simulink model "old_FMS"  (R2018b)
settings: configuration reference "FMS_config" (kept outside this file)
undefined symbols (not defined in the file): actuator_cmd, DiscIntNeverNeededParam, FMS_EXPORT, FMS_PARAM, mode, p_cmd, phi_cmd, psi_rate_cmd, q_cmd, r_cmd, reset, state, theta_cmd, throttle_cmd, timestamp, u_cmd, v_cmd, w_cmd
libraries: simulink x39, Rotation x2, Filter x1
(part 1 of 2)
settings Model: Creator=zouji  LastModifiedBy=zouji
settings ConfigSetRef: SourceLocation=Base Workspace

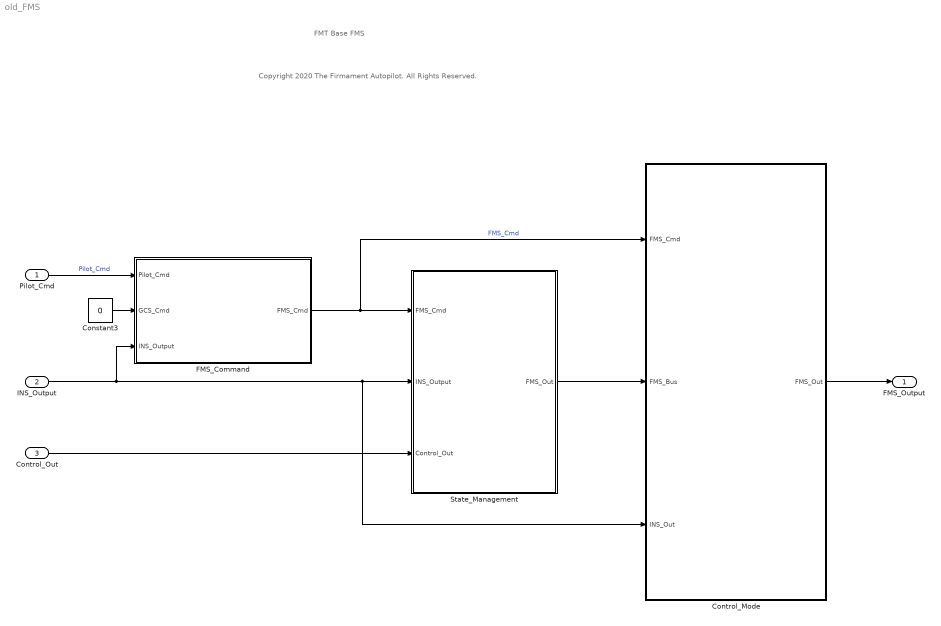
== system old_FMS ==
  note: FMT Base FMS
  note: Copyright 2020 The Firmament Autopilot. All Rights Reserved.
  Pilot_Cmd : Inport  OutDataTypeStr=Bus: Pilot_Cmd_Bus
  INS_Output : Inport  Port=2  OutDataTypeStr=Bus: INS_Out_Bus
  Control_Out : Inport  Port=3  OutDataTypeStr=Bus: Control_Out_Bus
  Constant3 : Constant  Value=0
  Control_Mode : Subsystem
  FMS_Command : Subsystem
  State_Management : Subsystem
  FMS_Output : Outport  OutDataTypeStr=Bus: FMS_Out_Bus
  wires:
  Control_Mode/1(FMS_Out) -> FMS_Output/1
  INS_Output/1 -> FMS_Command/3(INS_Output), Control_Mode/3(INS_Out), State_Management/2(INS_Output)
  Pilot_Cmd/1 -> FMS_Command/1(Pilot_Cmd)  "Pilot_Cmd"
  Constant3/1 -> FMS_Command/2(GCS_Cmd)
  FMS_Command/1(FMS_Cmd) -> Control_Mode/1(FMS_Cmd), State_Management/1(FMS_Cmd)  "FMS_Cmd"
  State_Management/1(FMS_Out) -> Control_Mode/2(FMS_Bus)
  Control_Out/1 -> State_Management/3(Control_Out)

== system old_FMS/Control_Mode ==
  FMS_Cmd : Inport
  FMS_Bus : Inport  Port=2
  INS_Out : Inport  Port=3
  Acro_Mode : Subsystem  TreatAsAtomicUnit=on
  Altitude_Hold_Mode : Subsystem  TreatAsAtomicUnit=on
  Bus Selector : BusSelector  OutputSignals=flag
  Bus Selector1 : BusSelector  OutputSignals=mode
  Manual_Mode : Subsystem  TreatAsAtomicUnit=on
  Merge : Merge  Inputs=5
  Mode_Logic : Stateflow chart  TreatAsAtomicUnit=on
  Position_Mode : Subsystem  TreatAsAtomicUnit=on
  Switch Case : SwitchCase  CaseConditions={2,3,4,5}
  Unknown_Mode : Subsystem  TreatAsAtomicUnit=on
  FMS_Out : Outport
  wires:
  INS_Out/1 -> Manual_Mode/2(INS_Out), Altitude_Hold_Mode/2(INS_Out), Position_Mode/2(INS_Out), Bus Selector/1
  FMS_Cmd/1 -> Bus Selector1/1, Manual_Mode/1(FMS_Cmd), Acro_Mode/2(FMS_Cmd), Altitude_Hold_Mode/1(FMS_Cmd), Position_Mode/1(FMS_Cmd)
  Switch Case/1 -> Position_Mode/Action
  Position_Mode/1(FMS_Out) -> Merge/1
  Switch Case/5 -> Unknown_Mode/Action
  Bus Selector/1 -> Mode_Logic/2(flag)  "<flag>"
  Merge/1 -> FMS_Out/1
  Unknown_Mode/1(FMS_Out) -> Merge/5
  FMS_Bus/1 -> Unknown_Mode/1(FMS_Bus), Acro_Mode/1(FMS_Bus), Manual_Mode/3(FMS_Bus), Altitude_Hold_Mode/3(FMS_Bus), Position_Mode/3(FMS_Bus)
  Bus Selector1/1 -> Mode_Logic/1(mode)  "<mode>"
  Mode_Logic/1(control_mode) -> Switch Case/1  "control_mode"
  Switch Case/2 -> Altitude_Hold_Mode/Action
  Altitude_Hold_Mode/1(FMS_Out) -> Merge/2
  Switch Case/3 -> Manual_Mode/Action
  Manual_Mode/1(FMS_Out) -> Merge/3
  Acro_Mode/1(FMS_Out) -> Merge/4
  Switch Case/4 -> Acro_Mode/Action

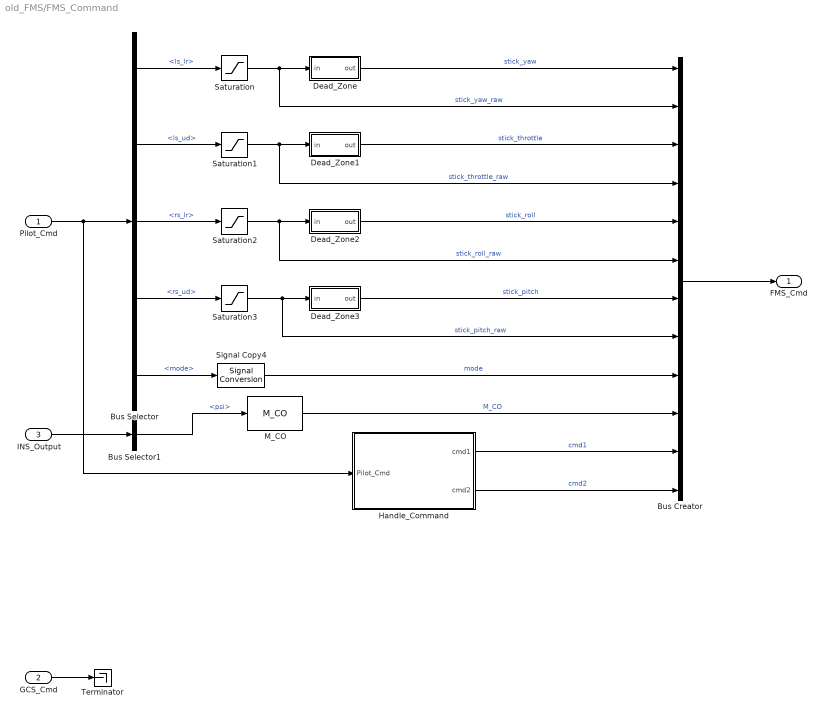
== system old_FMS/FMS_Command ==
  Pilot_Cmd : Inport
  GCS_Cmd : Inport  Port=2
  INS_Output : Inport  Port=3
  Bus Creator : BusCreator  Inputs=12
  Bus Selector : BusSelector  OutputSignals=ls_lr,ls_ud,rs_lr,rs_ud,mode
  Bus Selector1 : BusSelector  OutputSignals=psi
  Dead_Zone : Subsystem  mask{len=FMS_PARAM.StickDeadZone}
      mask prompts: len "Zone Half Length"
  Dead_Zone1 : Subsystem  mask{len=FMS_PARAM.StickDeadZone}
      mask prompts: len "Zone Half Length"
  Dead_Zone2 : Subsystem  mask{len=FMS_PARAM.StickDeadZone}
      mask prompts: len "Zone Half Length"
  Dead_Zone3 : Subsystem  mask{len=FMS_PARAM.StickDeadZone}
      mask prompts: len "Zone Half Length"
  Handle_Command : Subsystem
  M_CO : Rotation/M_CO  SystemSampleTime=-1
  Saturation{,1..3} (4 alike) : Saturate  UpperLimit=1  LowerLimit=-1
  Signal Copy4 : SignalConversion  OverrideOpt=off
  Terminator : Terminator
  FMS_Cmd : Outport
  wires:
  GCS_Cmd/1 -> Terminator/1
  Pilot_Cmd/1 -> Handle_Command/1(Pilot_Cmd), Bus Selector/1
  Bus Selector/1 -> Saturation/1  "<ls_lr>"
  Bus Selector/2 -> Saturation1/1  "<ls_ud>"
  Bus Selector/3 -> Saturation2/1  "<rs_lr>"
  Bus Selector/4 -> Saturation3/1  "<rs_ud>"
  Bus Selector/5 -> Signal Copy4/1  "<mode>"
  Saturation/1 -> Bus Creator/2, Dead_Zone/1(in)  "stick_yaw_raw"
  Saturation1/1 -> Bus Creator/4, Dead_Zone1/1(in)  "stick_throttle_raw"
  Saturation2/1 -> Bus Creator/6, Dead_Zone2/1(in)  "stick_roll_raw"
  Saturation3/1 -> Bus Creator/8, Dead_Zone3/1(in)  "stick_pitch_raw"
  Signal Copy4/1 -> Bus Creator/9  "mode"
  Bus Creator/1 -> FMS_Cmd/1
  Dead_Zone/1(out) -> Bus Creator/1  "stick_yaw"
  Dead_Zone1/1(out) -> Bus Creator/3  "stick_throttle"
  Dead_Zone2/1(out) -> Bus Creator/5  "stick_roll"
  Dead_Zone3/1(out) -> Bus Creator/7  "stick_pitch"
  INS_Output/1 -> Bus Selector1/1
  Bus Selector1/1 -> M_CO/1  "<psi>"
  M_CO/1 -> Bus Creator/10  "M_CO"
  Handle_Command/1(cmd1) -> Bus Creator/11  "cmd1"
  Handle_Command/2(cmd2) -> Bus Creator/12  "cmd2"

== system old_FMS/State_Management ==
  FMS_Cmd : Inport
  INS_Output : Inport  Port=2
  Control_Out : Inport  Port=3
  Arm_Event : Subsystem
  "Arm_Prerequisite " : Subsystem
      settings: MinAlgLoopOccurrences=on
  Bus Assignment : BusAssignment  AssignedSignals=actuator_cmd,state,reset,timestamp
  Bus Selector : BusSelector  OutputSignals=cmd1.cmd1_force_disarm,cmd2.cmd2_test_motor
  Compare To Constant : simulink/Logic and Bit Operations/Compare To Constant  relop=<  const=2  OutDataTypeStr=uint8
  Constant : Constant  Value=0  OutDataTypeStr=Bus: FMS_Out_Bus
  Delay : Delay  DelayLength=1
  State_Logic : Stateflow chart  TreatAsAtomicUnit=on
  Subsystem : Subsystem
  timestamp : Subsystem  mask{sample_time=FMS_EXPORT.period}
      mask prompts: sample_time "sample time (ms)"
  FMS_Out : Outport
  wires:
  Constant/1 -> Bus Assignment/1
  Bus Assignment/1 -> FMS_Out/1
  Arm_Event/2(disarm_event) -> State_Logic/4(Disarm_Event)
  Arm_Event/1(arm_event) -> State_Logic/3(Arm_Event)
  FMS_Cmd/1 -> Bus Selector/1, Arm_Event/2(FMS_Cmd)
  "Arm_Prerequisite "/2(Disarm_Allowed) -> State_Logic/2(Disarm_Allowed)
  "Arm_Prerequisite "/1(Arm_Allowed) -> State_Logic/1(Arm_Allowed)
  INS_Output/1 -> Arm_Event/1(INS_Output), "Arm_Prerequisite "/1(INS_Output)
  State_Logic/1(PWM_Cmd) -> Subsystem/1(pwm_in)
  Subsystem/1(pwm_out) -> Bus Assignment/2
  State_Logic/2(State) -> Delay/1, Compare To Constant/1, Bus Assignment/3
  Compare To Constant/1 -> Bus Assignment/4
  Arm_Event/3(Stick_Throttle) -> State_Logic/5(Stick_Throttle)
  timestamp/1(timestamp_ms) -> Bus Assignment/5
  Control_Out/1 -> Arm_Event/3(Control_Out)
  Delay/1 -> Arm_Event/4(State)
  Bus Selector/1 -> State_Logic/6(Force_Disarm)  "<cmd1_force_disarm>"
  Bus Selector/2 -> State_Logic/7(Test_Motor)  "<cmd2_test_motor>"

== system old_FMS/Control_Mode/Acro_Mode ==
  FMS_Bus : Inport
  FMS_Cmd : Inport  Port=2
  Action Port : ActionPort  InitializeStates=reset  ActionType=case
  Bus Assignment : BusAssignment  AssignedSignals=mode,throttle_cmd,p_cmd,q_cmd,r_cmd
  Command_Generator : Subsystem
  Constant : Constant  Value=5  OutDataTypeStr=Inherit: Inherit via back propagation
  FMS_Out : Outport
  wires:
  Bus Assignment/1 -> FMS_Out/1
  Constant/1 -> Bus Assignment/2
  FMS_Bus/1 -> Bus Assignment/1
  Command_Generator/1(throttle_cmd) -> Bus Assignment/3
  Command_Generator/2(p_cmd_radPs) -> Bus Assignment/4
  Command_Generator/3(q_cmd_radPs) -> Bus Assignment/5
  Command_Generator/4(r_cmd_radPs) -> Bus Assignment/6
  FMS_Cmd/1 -> Command_Generator/1(FMS_Cmd)

== system old_FMS/Control_Mode/Altitude_Hold_Mode ==
  FMS_Cmd : Inport
  INS_Out : Inport  Port=2
  FMS_Bus : Inport  Port=3
  Action Port : ActionPort  InitializeStates=reset  ActionType=case
  Bus Assignment : BusAssignment  AssignedSignals=mode,phi_cmd,theta_cmd,w_cmd,psi_rate_cmd
  Command_Generator : Subsystem
  Constant : Constant  Value=3  OutDataTypeStr=Inherit: Inherit via back propagation
  FMS_Out : Outport
  wires:
  FMS_Cmd/1 -> Command_Generator/3(FMS_Cmd)
  FMS_Bus/1 -> Command_Generator/1(FMS_Out), Bus Assignment/1
  Constant/1 -> Bus Assignment/2
  INS_Out/1 -> Command_Generator/2(INS_Out)
  Bus Assignment/1 -> FMS_Out/1
  Command_Generator/3(w_cmd_C_mPs) -> Bus Assignment/5
  Command_Generator/4(psi_rate_cmd_radPs) -> Bus Assignment/6
  Command_Generator/1(phi_cmd_rad) -> Bus Assignment/3
  Command_Generator/2(theta_cmd_rad) -> Bus Assignment/4

== system old_FMS/Control_Mode/Manual_Mode ==
  FMS_Cmd : Inport
  INS_Out : Inport  Port=2
  FMS_Bus : Inport  Port=3
  Action Port : ActionPort  InitializeStates=reset  ActionType=case
  Bus Assignment : BusAssignment  AssignedSignals=mode,throttle_cmd,phi_cmd,theta_cmd,psi_rate_cmd
  Command_Generator : Subsystem
  Constant : Constant  Value=4  OutDataTypeStr=Inherit: Inherit via back propagation
  FMS_Out : Outport
  wires:
  Bus Assignment/1 -> FMS_Out/1
  INS_Out/1 -> Command_Generator/2(INS_Out)
  Constant/1 -> Bus Assignment/2
  FMS_Bus/1 -> Command_Generator/1(FMS_Out), Bus Assignment/1
  FMS_Cmd/1 -> Command_Generator/3(FMS_Cmd)
  Command_Generator/1(throttle_cmd) -> Bus Assignment/3
  Command_Generator/2(phi_cmd_rad) -> Bus Assignment/4
  Command_Generator/3(theta_cmd_rad) -> Bus Assignment/5
  Command_Generator/4(psi_rate_cmd_radPs) -> Bus Assignment/6

== system old_FMS/Control_Mode/Position_Mode ==
  FMS_Cmd : Inport
  INS_Out : Inport  Port=2
  FMS_Bus : Inport  Port=3
  Action Port : ActionPort  InitializeStates=reset  ActionType=case
  Bus Assignment : BusAssignment  AssignedSignals=mode,u_cmd,v_cmd,w_cmd,psi_rate_cmd
  Command_Generator : Subsystem
  Constant : Constant  Value=2  OutDataTypeStr=Inherit: Inherit via back propagation
  FMS_Out : Outport
  wires:
  FMS_Cmd/1 -> Command_Generator/3(FMS_Cmd)
  FMS_Bus/1 -> Command_Generator/1(FMS_Out), Bus Assignment/1
  Constant/1 -> Bus Assignment/2
  INS_Out/1 -> Command_Generator/2(INS_Out)
  Bus Assignment/1 -> FMS_Out/1
  Command_Generator/1(u_cmd_C_mPs) -> Bus Assignment/3
  Command_Generator/2(v_cmd_C_mPs) -> Bus Assignment/4
  Command_Generator/3(w_cmd_C_mPs) -> Bus Assignment/5
  Command_Generator/4(psi_rate_cmd_radPs) -> Bus Assignment/6

== system old_FMS/Control_Mode/Unknown_Mode ==
  FMS_Bus : Inport
  Action Port : ActionPort  InitializeStates=reset  ActionType=default
  Bus Assignment : BusAssignment  AssignedSignals=mode,reset
  Constant1 : Constant  Value=0  OutDataTypeStr=Inherit: Inherit via back propagation
  Constant2 : Constant  OutDataTypeStr=Inherit: Inherit via back propagation
  FMS_Out : Outport
  wires:
  Bus Assignment/1 -> FMS_Out/1
  FMS_Bus/1 -> Bus Assignment/1
  Constant1/1 -> Bus Assignment/2
  Constant2/1 -> Bus Assignment/3

== system old_FMS/FMS_Command/Dead_Zone ==
  in : Inport
  Add : Sum
  Constant : Constant  Value=len  OutDataTypeStr=single
  Dead Zone : DeadZone  LowerValue=-len  UpperValue=len  SaturateOnIntegerOverflow=on
  Multiply : Product
  Sign : Signum
  out : Outport
  wires:
  in/1 -> Dead Zone/1
  Dead Zone/1 -> Sign/1, Add/1
  Sign/1 -> Multiply/1
  Constant/1 -> Multiply/2
  Multiply/1 -> Add/2
  Add/1 -> out/1

== system old_FMS/FMS_Command/Dead_Zone1 ==
  in : Inport
  Add : Sum
  Constant : Constant  Value=len  OutDataTypeStr=single
  Dead Zone : DeadZone  LowerValue=-len  UpperValue=len  SaturateOnIntegerOverflow=on
  Multiply : Product
  Sign : Signum
  out : Outport
  wires:
  Add/1 -> out/1
  Multiply/1 -> Add/2
  Constant/1 -> Multiply/2
  Sign/1 -> Multiply/1
  Dead Zone/1 -> Add/1, Sign/1
  in/1 -> Dead Zone/1

== system old_FMS/FMS_Command/Dead_Zone2 ==
  in : Inport
  Add : Sum
  Constant : Constant  Value=len  OutDataTypeStr=single
  Dead Zone : DeadZone  LowerValue=-len  UpperValue=len  SaturateOnIntegerOverflow=on
  Multiply : Product
  Sign : Signum
  out : Outport
  wires:
  in/1 -> Dead Zone/1
  Dead Zone/1 -> Sign/1, Add/1
  Sign/1 -> Multiply/1
  Constant/1 -> Multiply/2
  Multiply/1 -> Add/2
  Add/1 -> out/1

== system old_FMS/FMS_Command/Dead_Zone3 ==
  in : Inport
  Add : Sum
  Constant : Constant  Value=len  OutDataTypeStr=single
  Dead Zone : DeadZone  LowerValue=-len  UpperValue=len  SaturateOnIntegerOverflow=on
  Multiply : Product
  Sign : Signum
  out : Outport
  wires:
  Add/1 -> out/1
  Multiply/1 -> Add/2
  Constant/1 -> Multiply/2
  Sign/1 -> Multiply/1
  Dead Zone/1 -> Add/1, Sign/1
  in/1 -> Dead Zone/1

== system old_FMS/FMS_Command/Handle_Command ==
  Pilot_Cmd : Inport
  Bus Creator : BusCreator  Inputs=1
  Bus Creator1 : BusCreator  Inputs=1
  Bus Selector1 : BusSelector  OutputSignals=cmd_2
  Bus Selector2 : BusSelector  OutputSignals=cmd_1
  Compare To Constant : simulink/Logic and Bit Operations/Compare To Constant  relop===  const=1000  OutDataTypeStr=boolean
  Compare To Constant3 : simulink/Logic and Bit Operations/Compare To Constant  relop===  const=2000  OutDataTypeStr=boolean
  Detect Increase : simulink/Logic and Bit Operations/Detect Increase  vinit=0.0  OutDataTypeStr=boolean
  cmd1 : Outport
  cmd2 : Outport  Port=2
  wires:
  Bus Selector2/1 -> Compare To Constant/1  "<cmd_1>"
  Compare To Constant/1 -> Detect Increase/1
  Pilot_Cmd/1 -> Bus Selector1/1, Bus Selector2/1
  Detect Increase/1 -> Bus Creator/1  "cmd1_force_disarm"
  Bus Creator/1 -> cmd1/1
  Bus Selector1/1 -> Compare To Constant3/1  "<cmd_2>"
  Compare To Constant3/1 -> Bus Creator1/1  "cmd2_test_motor"
  Bus Creator1/1 -> cmd2/1

== system old_FMS/State_Management/Arm_Event ==
  INS_Output : Inport
  FMS_Cmd : Inport  Port=2
  Control_Out : Inport  Port=3
  State : Inport  Port=4
  Arm_Event : Stateflow chart  TreatAsAtomicUnit=on
  Bus Selector : BusSelector  OutputSignals=stick_roll,stick_pitch,stick_throttle_raw
  Disarm_Event : Stateflow chart  TreatAsAtomicUnit=on
  Onground_Check : Subsystem
  arm_event : Outport
  disarm_event : Outport  Port=2
  Stick_Throttle : Outport  Port=3
  wires:
  Arm_Event/1(arm_event) -> arm_event/1
  FMS_Cmd/1 -> Bus Selector/1
  Bus Selector/1 -> Arm_Event/1(stick_roll)  "<stick_roll>"
  Bus Selector/2 -> Arm_Event/2(stick_pitch)  "<stick_pitch>"
  Bus Selector/3 -> Stick_Throttle/1, Arm_Event/3(stick_throttle)  "<stick_throttle_raw>"
  Disarm_Event/1(disarm_event) -> disarm_event/1  "disarm_event"
  INS_Output/1 -> Onground_Check/1(INS_Output)
  Control_Out/1 -> Onground_Check/2(Control_Out)
  Onground_Check/1(on_ground) -> Disarm_Event/1(on_ground)  "on_ground"
  State/1 -> Disarm_Event/2(state)

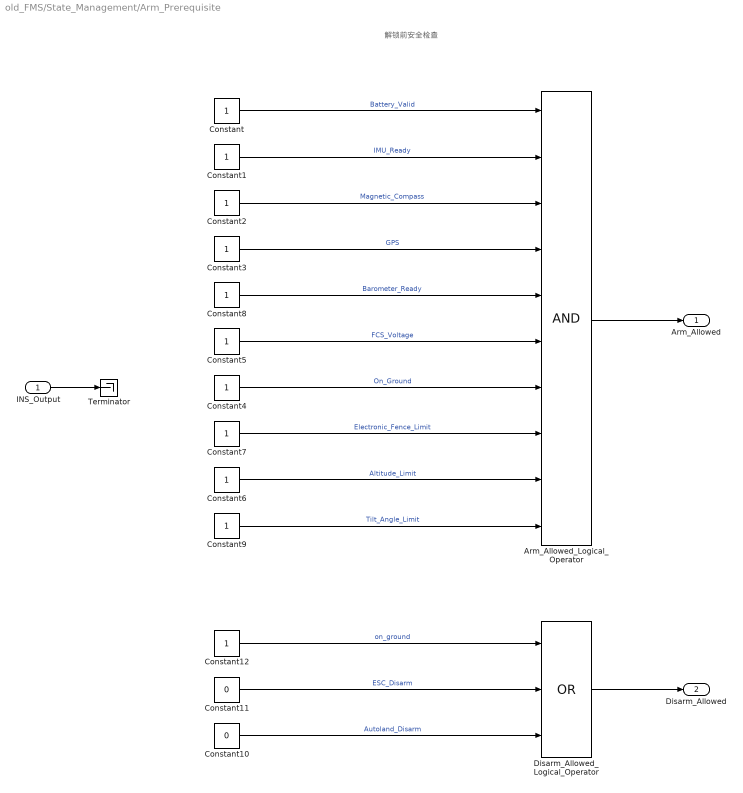
== system old_FMS/State_Management/Arm_Prerequisite  ==
  note: 解锁前安全检查
  INS_Output : Inport
  Arm_Allowed_Logical_Operator : Logic  Inputs=10  AllPortsSameDT=off  OutDataTypeStr=boolean
  Constant{,1..9,12} (11 alike) : Constant  OutDataTypeStr=boolean
  Constant10 : Constant  Value=0  OutDataTypeStr=boolean
  Constant11 : Constant  Value=0  OutDataTypeStr=boolean
  Disarm_Allowed_Logical_Operator : Logic  Operator=OR  Inputs=3  AllPortsSameDT=off  OutDataTypeStr=boolean
  Terminator : Terminator
  Arm_Allowed : Outport
  Disarm_Allowed : Outport  Port=2
  wires:
  Constant/1 -> Arm_Allowed_Logical_Operator/1  "Battery_Valid"
  Arm_Allowed_Logical_Operator/1 -> Arm_Allowed/1
  Constant1/1 -> Arm_Allowed_Logical_Operator/2  "IMU_Ready"
  Constant2/1 -> Arm_Allowed_Logical_Operator/3  "Magnetic_Compass"
  Constant3/1 -> Arm_Allowed_Logical_Operator/4  "GPS"
  Constant4/1 -> Arm_Allowed_Logical_Operator/7  "On_Ground"
  Constant5/1 -> Arm_Allowed_Logical_Operator/6  "FCS_Voltage"
  Constant6/1 -> Arm_Allowed_Logical_Operator/9  "Altitude_Limit"
  Constant7/1 -> Arm_Allowed_Logical_Operator/8  "Electronic_Fence_Limit"
  Constant8/1 -> Arm_Allowed_Logical_Operator/5  "Barometer_Ready"
  Constant9/1 -> Arm_Allowed_Logical_Operator/10  "Tilt_Angle_Limit"
  Disarm_Allowed_Logical_Operator/1 -> Disarm_Allowed/1
  Constant10/1 -> Disarm_Allowed_Logical_Operator/3  "Autoland_Disarm"
  Constant11/1 -> Disarm_Allowed_Logical_Operator/2  "ESC_Disarm"
  INS_Output/1 -> Terminator/1
  Constant12/1 -> Disarm_Allowed_Logical_Operator/1  "on_ground"

== system old_FMS/State_Management/Subsystem ==
  pwm_in : Inport
  Multiply : Product  OutDataTypeStr=uint16
  One : Constant  Value=ones(16,1)  OutDataTypeStr=uint16
  pwm_out : Outport
  wires:
  pwm_in/1 -> Multiply/2
  One/1 -> Multiply/1
  Multiply/1 -> pwm_out/1

== system old_FMS/State_Management/timestamp ==
  Constant : Constant  Value=sample_time  OutDataTypeStr=uint32
  Data Type Conversion : DataTypeConversion  OutDataTypeStr=uint32
  Discrete-Time Integrator : DiscreteIntegrator  IntegratorMethod=Accumulation: Forward Euler  SampleTime=-1  ICPrevOutput=DiscIntNeverNeededParam  ICPrevScaledInput=DiscIntNeverNeededParam
  timestamp_ms : Outport
  wires:
  Discrete-Time Integrator/1 -> Data Type Conversion/1
  Constant/1 -> Discrete-Time Integrator/1
  Data Type Conversion/1 -> timestamp_ms/1

== system old_FMS/Control_Mode/Acro_Mode/Command_Generator ==
  FMS_Cmd : Inport
  Angel_Rate_Command : Subsystem
  Throttle_Command : Subsystem
  throttle_cmd : Outport
  p_cmd_radPs : Outport  Port=2
  q_cmd_radPs : Outport  Port=3
  r_cmd_radPs : Outport  Port=4
  wires:
  Angel_Rate_Command/1(p_cmd_radPs) -> p_cmd_radPs/1
  FMS_Cmd/1 -> Throttle_Command/1(FMS_Cmd), Angel_Rate_Command/1(FMS_Cmd)
  Throttle_Command/1(throttle_cmd) -> throttle_cmd/1
  Angel_Rate_Command/3(r_cmd_radPs) -> r_cmd_radPs/1
  Angel_Rate_Command/2(q_cmd_radPs) -> q_cmd_radPs/1

== system old_FMS/Control_Mode/Altitude_Hold_Mode/Command_Generator ==
  FMS_Out : Inport
  INS_Out : Inport  Port=2
  FMS_Cmd : Inport  Port=3
  Attitude_Command : Subsystem
  Psi_Rate_Command : Subsystem
  Vel_Command : Subsystem
  phi_cmd_rad : Outport
  theta_cmd_rad : Outport  Port=2
  w_cmd_C_mPs : Outport  Port=3
  psi_rate_cmd_radPs : Outport  Port=4
  wires:
  FMS_Cmd/1 -> Attitude_Command/1(FMS_Cmd), Psi_Rate_Command/1(FMS_Cmd), Vel_Command/1(FMS_Cmd)
  INS_Out/1 -> Vel_Command/2(INS_Out), Psi_Rate_Command/3(INS_Out)
  Vel_Command/1(vel_w_cmd_C_mPs) -> w_cmd_C_mPs/1
  Psi_Rate_Command/1(psi_rate_cmd_radPs) -> psi_rate_cmd_radPs/1
  Attitude_Command/1(phi_cmd_rad) -> phi_cmd_rad/1
  Attitude_Command/2(theta_cmd_rad) -> theta_cmd_rad/1
  FMS_Out/1 -> Psi_Rate_Command/2(FMS_Out)

== system old_FMS/Control_Mode/Manual_Mode/Command_Generator ==
  FMS_Out : Inport
  INS_Out : Inport  Port=2
  FMS_Cmd : Inport  Port=3
  Attitude_Command : Subsystem
  Psi_Rate_Command : Subsystem
  Throttle_Command : Subsystem
  throttle_cmd : Outport
  phi_cmd_rad : Outport  Port=2
  theta_cmd_rad : Outport  Port=3
  psi_rate_cmd_radPs : Outport  Port=4
  wires:
  Attitude_Command/2(theta_cmd_rad) -> theta_cmd_rad/1
  Attitude_Command/1(phi_cmd_rad) -> phi_cmd_rad/1
  Psi_Rate_Command/1(psi_rate_cmd_radPs) -> psi_rate_cmd_radPs/1
  INS_Out/1 -> Psi_Rate_Command/3(INS_Out)
  FMS_Cmd/1 -> Throttle_Command/1(FMS_Cmd), Psi_Rate_Command/1(FMS_Cmd), Attitude_Command/1(FMS_Cmd)
  Throttle_Command/1(throttle_cmd) -> throttle_cmd/1
  FMS_Out/1 -> Psi_Rate_Command/2(FMS_Out)

== system old_FMS/Control_Mode/Position_Mode/Command_Generator ==
  FMS_Out : Inport
  INS_Out : Inport  Port=2
  FMS_Cmd : Inport  Port=3
  Demux : Demux  Outputs=3
  Psi_Rate_Command1 : Subsystem
  Vel_Command : Subsystem
  u_cmd_C_mPs : Outport
  v_cmd_C_mPs : Outport  Port=2
  w_cmd_C_mPs : Outport  Port=3
  psi_rate_cmd_radPs : Outport  Port=4
  wires:
  FMS_Cmd/1 -> Psi_Rate_Command1/1(FMS_Cmd), Vel_Command/1(FMS_Cmd)
  INS_Out/1 -> Psi_Rate_Command1/3(INS_Out), Vel_Command/2(INS_Out)
  Vel_Command/1(vel_cmd_C_mPs) -> Demux/1
  Demux/1 -> u_cmd_C_mPs/1
  Demux/2 -> v_cmd_C_mPs/1
  Demux/3 -> w_cmd_C_mPs/1
  Psi_Rate_Command1/1(psi_rate_cmd_radPs) -> psi_rate_cmd_radPs/1
  FMS_Out/1 -> Psi_Rate_Command1/2(FMS_Out)

== system old_FMS/State_Management/Arm_Event/Onground_Check ==
  INS_Output : Inport
  Control_Out : Inport  Port=2
  Bus Selector1 : BusSelector  OutputSignals=actuator_cmd
  Bus Selector2 : BusSelector  OutputSignals=quat
  Bus Selector3 : BusSelector  OutputSignals=ax,ay,az
  Compare To Constant : simulink/Logic and Bit Operations/Compare To Constant  relop=<  const=1200  OutDataTypeStr=boolean
  Constant : Constant  Value=4  OutDataTypeStr=uint16
  Divide : Product  Inputs=*/
  Interval Test : simulink/Logic and Bit Operations/Interval Test  IntervalClosedRight=on  uplimit=-9.806+1  IntervalClosedLeft=on  lowlimit=-9.806-1  OutDataTypeStr=boolean
  LPF : Filter/LPF  T=0.1
  Logical Operator1 : Logic  AllPortsSameDT=off  OutDataTypeStr=boolean
  Matrix Concatenate3 : Concatenate  NumInputs=3  ConcatenateDimension=2
  Multiply : Product  Multiplication=Matrix(*)
  Quat_to_M_OB : Rotation/Quat_to_M_OB  SystemSampleTime=-1
  Selector : Selector  InputPortWidth=16  IndexOptions=Index vector (dialog)  Indices=[1:4]  OutputSizes=1
  Selector1 : Selector  InputPortWidth=3  IndexOptions=Index vector (dialog)  Indices=3  OutputSizes=1
  Sum of Elements : Sum  Inputs=+
  on_ground : Outport
  wires:
  Multiply/1 -> Selector1/1
  Quat_to_M_OB/1 -> Multiply/1
  Bus Selector3/2 -> Matrix Concatenate3/2  "<ay>"
  Compare To Constant/1 -> Logical Operator1/2
  Bus Selector3/3 -> Matrix Concatenate3/3  "<az>"
  Matrix Concatenate3/1 -> Multiply/2
  Bus Selector1/1 -> Selector/1  "<actuator_cmd>"
  Bus Selector3/1 -> Matrix Concatenate3/1  "<ax>"
  Bus Selector2/1 -> Quat_to_M_OB/1  "<quat>"
  Selector/1 -> Sum of Elements/1
  INS_Output/1 -> Bus Selector2/1, Bus Selector3/1
  Logical Operator1/1 -> on_ground/1
  Control_Out/1 -> Bus Selector1/1
  Selector1/1 -> LPF/1
  Interval Test/1 -> Logical Operator1/1
  Sum of Elements/1 -> Divide/1
  Constant/1 -> Divide/2
  Divide/1 -> Compare To Constant/1
  LPF/1 -> Interval Test/1

== system old_FMS/Control_Mode/Acro_Mode/Command_Generator/Angel_Rate_Command ==
  FMS_Cmd : Inport
  Bus Selector : BusSelector  OutputSignals=stick_roll_raw,stick_pitch_raw,stick_yaw_raw
  Gain : Gain  Gain=pi/3  OutDataTypeStr=Inherit: Same as input
  Gain1 : Gain  Gain=-pi/3  OutDataTypeStr=Inherit: Same as input
  Gain2 : Gain  Gain=pi/3  OutDataTypeStr=Inherit: Same as input
  p_cmd_radPs : Outport
  q_cmd_radPs : Outport  Port=2
  r_cmd_radPs : Outport  Port=3
  wires:
  Bus Selector/2 -> Gain1/1  "<stick_pitch_raw>"
  Bus Selector/1 -> Gain/1  "<stick_roll_raw>"
  FMS_Cmd/1 -> Bus Selector/1
  Gain/1 -> p_cmd_radPs/1
  Gain1/1 -> q_cmd_radPs/1
  Bus Selector/3 -> Gain2/1  "<stick_yaw_raw>"
  Gain2/1 -> r_cmd_radPs/1

== system old_FMS/Control_Mode/Acro_Mode/Command_Generator/Throttle_Command ==
  FMS_Cmd : Inport
  Add : Sum
  Bus Selector : BusSelector  OutputSignals=stick_throttle_raw
  Constant : Constant  OutDataTypeStr=single
  Constant1 : Constant  Value=1000  OutDataTypeStr=uint32
  Gain : Gain  Gain=500  OutDataTypeStr=uint32
  Sum : Sum  Inputs=|++
  throttle_cmd : Outport
  wires:
  FMS_Cmd/1 -> Bus Selector/1
  Gain/1 -> Add/1
  Bus Selector/1 -> Sum/1  "<stick_throttle_raw>"
  Add/1 -> throttle_cmd/1
  Constant/1 -> Sum/2
  Sum/1 -> Gain/1
  Constant1/1 -> Add/2

== system old_FMS/Control_Mode/Altitude_Hold_Mode/Command_Generator/Attitude_Command ==
  FMS_Cmd : Inport
  Bus Selector : BusSelector  OutputSignals=stick_roll_raw,stick_pitch_raw
  Gain : Gain  Gain=FMS_PARAM.ROLL_PITCH_LIM
  Gain1 : Gain  Gain=-FMS_PARAM.ROLL_PITCH_LIM
  Phi_CMD_TD : Subsystem
  Thera_CMD_TD : Subsystem
  phi_cmd_rad : Outport
  theta_cmd_rad : Outport  Port=2
  wires:
  Gain/1 -> Phi_CMD_TD/1(v)
  FMS_Cmd/1 -> Bus Selector/1
  Bus Selector/1 -> Gain/1  "<stick_roll_raw>"
  Bus Selector/2 -> Gain1/1  "<stick_pitch_raw>"
  Gain1/1 -> Thera_CMD_TD/1(v)
  Phi_CMD_TD/1(v1) -> phi_cmd_rad/1
  Thera_CMD_TD/1(v1) -> theta_cmd_rad/1

== system old_FMS/Control_Mode/Altitude_Hold_Mode/Command_Generator/Psi_Rate_Command ==
  FMS_Cmd : Inport
  FMS_Out : Inport  Port=2
  INS_Out : Inport  Port=3
  Bus Selector : BusSelector  OutputSignals=state
  Compare To Constant : simulink/Logic and Bit Operations/Compare To Constant  relop===  const=2  OutDataTypeStr=boolean
  Compare To Constant1 : simulink/Logic and Bit Operations/Compare To Constant  relop===  const=2  OutDataTypeStr=boolean
  Detect Increase : simulink/Logic and Bit Operations/Detect Increase  vinit=0.0  OutDataTypeStr=boolean
  Detect Increase1 : simulink/Logic and Bit Operations/Detect Increase  vinit=0.0  OutDataTypeStr=boolean
  Heading_Control : Subsystem
  Heading_Rate_Map : Subsystem
  Logical Operator : Logic  Operator=OR  AllPortsSameDT=off  OutDataTypeStr=boolean
  Motion_State : Stateflow chart  TreatAsAtomicUnit=on
  Psi_rate_cmd_TD : Subsystem
  Saturation1 : Saturate  UpperLimit=FMS_PARAM.YAW_RATE_LIM  LowerLimit=-FMS_PARAM.YAW_RATE_LIM
  Switch : Switch  Criteria=u2 > Threshold
  move_check : Subsystem
  psi_rate : Subsystem
  psi_rate_cmd_radPs : Outport
  wires:
  Saturation1/1 -> psi_rate_cmd_radPs/1
  Switch/1 -> Psi_rate_cmd_TD/1(v)
  INS_Out/1 -> Heading_Control/2(INS_Out), psi_rate/1(INS_Out)
  move_check/1(move_cmd) -> Motion_State/1(move_cmd)
  psi_rate/1(heading_rate) -> Motion_State/2(heading_rate)
  Compare To Constant/1 -> Switch/2, Detect Increase/1
  FMS_Cmd/1 -> Heading_Rate_Map/2(FMS_Cmd), move_check/1(FMS_Cmd)
  Heading_Rate_Map/1(psi_rate_cmd_radPs) -> Switch/3
  Motion_State/1(state) -> Compare To Constant/1, Heading_Rate_Map/1(state)  "alt_mode_psi_state"
  Logical Operator/1 -> Heading_Control/1(update)
  Heading_Control/1(psi_rate_cmd_radPs) -> Switch/1
  FMS_Out/1 -> Bus Selector/1
  Bus Selector/1 -> Compare To Constant1/1  "<state>"
  Compare To Constant1/1 -> Detect Increase1/1
  Detect Increase1/1 -> Logical Operator/1  "just_arm"
  Detect Increase/1 -> Logical Operator/2
  Psi_rate_cmd_TD/1(v1) -> Saturation1/1

== system old_FMS/Control_Mode/Altitude_Hold_Mode/Command_Generator/Vel_Command ==
  FMS_Cmd : Inport
  INS_Out : Inport  Port=2
  Motion_State : Subsystem
  Saturation : Saturate  UpperLimit=FMS_PARAM.VEL_Z_LIM  LowerLimit=-FMS_PARAM.VEL_Z_LIM
  Subsystem1 : Subsystem
  line_speed : Subsystem
  move_check : Subsystem
  vel_w_cmd_C_mPs : Outport
  wires:
  Saturation/1 -> vel_w_cmd_C_mPs/1
  Subsystem1/1(vel_w_cmd_C_mPs) -> Saturation/1
  FMS_Cmd/1 -> Subsystem1/1(FMS_Cmd), move_check/1(FMS_Cmd)
  INS_Out/1 -> Subsystem1/3(INS_Out), line_speed/1(INS_Out)
  move_check/1(move_cmd) -> Motion_State/1(move_cmd)
  line_speed/1(vz) -> Motion_State/2(vz)
  Motion_State/1(motion_state) -> Subsystem1/2(motion_state)

== system old_FMS/Control_Mode/Manual_Mode/Command_Generator/Attitude_Command ==
  FMS_Cmd : Inport
  Bus Selector : BusSelector  OutputSignals=stick_roll_raw,stick_pitch_raw
  Gain1 : Gain  Gain=-FMS_PARAM.ROLL_PITCH_LIM
  Gain2 : Gain  Gain=FMS_PARAM.ROLL_PITCH_LIM
  Phi_CMD_TD : Subsystem
  Theta_CMD_TD : Subsystem
  phi_cmd_rad : Outport
  theta_cmd_rad : Outport  Port=2
  wires:
  Bus Selector/2 -> Gain1/1  "<stick_pitch_raw>"
  Bus Selector/1 -> Gain2/1  "<stick_roll_raw>"
  FMS_Cmd/1 -> Bus Selector/1
  Gain2/1 -> Phi_CMD_TD/1(v)
  Gain1/1 -> Theta_CMD_TD/1(v)
  Phi_CMD_TD/1(v1) -> phi_cmd_rad/1
  Theta_CMD_TD/1(v1) -> theta_cmd_rad/1

== system old_FMS/Control_Mode/Manual_Mode/Command_Generator/Psi_Rate_Command ==
  FMS_Cmd : Inport
  FMS_Out : Inport  Port=2
  INS_Out : Inport  Port=3
  Bus Selector : BusSelector  OutputSignals=state
  Compare To Constant : simulink/Logic and Bit Operations/Compare To Constant  relop===  const=2  OutDataTypeStr=boolean
  Compare To Constant1 : simulink/Logic and Bit Operations/Compare To Constant  relop===  const=2  OutDataTypeStr=boolean
  Detect Increase : simulink/Logic and Bit Operations/Detect Increase  vinit=0.0  OutDataTypeStr=boolean
  Detect Increase1 : simulink/Logic and Bit Operations/Detect Increase  vinit=0.0  OutDataTypeStr=boolean
  Heading_Control : Subsystem
  Heading_Rate_Map : Subsystem
  Logical Operator : Logic  Operator=OR  AllPortsSameDT=off  OutDataTypeStr=boolean
  Motion_State : Stateflow chart  TreatAsAtomicUnit=on
  Saturation1 : Saturate  UpperLimit=FMS_PARAM.YAW_RATE_LIM  LowerLimit=-FMS_PARAM.YAW_RATE_LIM
  Switch : Switch  Criteria=u2 > Threshold
  move_check : Subsystem
  psi_rate : Subsystem
  psi_rate_cmd_radPs : Outport
  wires:
  Heading_Control/1(psi_rate_cmd_radPs) -> Switch/1
  Detect Increase/1 -> Logical Operator/2
  Motion_State/1(state) -> Compare To Constant/1, Heading_Rate_Map/1(state)  "manual_mode_psi_state"
  Heading_Rate_Map/1(psi_rate_cmd_radPs) -> Switch/3
  FMS_Cmd/1 -> move_check/1(FMS_Cmd), Heading_Rate_Map/2(FMS_Cmd)
  Compare To Constant/1 -> Switch/2, Detect Increase/1
  psi_rate/1(heading_rate) -> Motion_State/2(heading_rate)
  move_check/1(move_cmd) -> Motion_State/1(move_cmd)
  INS_Out/1 -> psi_rate/1(INS_Out), Heading_Control/2(INS_Out)
  Switch/1 -> Saturation1/1
  Saturation1/1 -> psi_rate_cmd_radPs/1
  FMS_Out/1 -> Bus Selector/1
  Bus Selector/1 -> Compare To Constant1/1  "<state>"
  Compare To Constant1/1 -> Detect Increase1/1
  Logical Operator/1 -> Heading_Control/1(update)
  Detect Increase1/1 -> Logical Operator/1  "just_arm"

== system old_FMS/Control_Mode/Manual_Mode/Command_Generator/Throttle_Command ==
  FMS_Cmd : Inport
  Add : Sum
  Bus Selector : BusSelector  OutputSignals=stick_throttle_raw
  Constant : Constant  OutDataTypeStr=single
  Constant1 : Constant  Value=1000  OutDataTypeStr=uint32
  Gain : Gain  Gain=500  OutDataTypeStr=uint32
  Sum : Sum  Inputs=|++
  throttle_cmd : Outport
  wires:
  FMS_Cmd/1 -> Bus Selector/1
  Gain/1 -> Add/1
  Bus Selector/1 -> Sum/1  "<stick_throttle_raw>"
  Add/1 -> throttle_cmd/1
  Constant/1 -> Sum/2
  Sum/1 -> Gain/1
  Constant1/1 -> Add/2

== system old_FMS/Control_Mode/Position_Mode/Command_Generator/Psi_Rate_Command1 ==
  FMS_Cmd : Inport
  FMS_Out : Inport  Port=2
  INS_Out : Inport  Port=3
  Bus Selector : BusSelector  OutputSignals=state
  Compare To Constant : simulink/Logic and Bit Operations/Compare To Constant  relop===  const=2  OutDataTypeStr=boolean
  Compare To Constant1 : simulink/Logic and Bit Operations/Compare To Constant  relop===  const=2  OutDataTypeStr=boolean
  Detect Increase : simulink/Logic and Bit Operations/Detect Increase  vinit=0.0  OutDataTypeStr=boolean
  Detect Increase1 : simulink/Logic and Bit Operations/Detect Increase  vinit=0.0  OutDataTypeStr=boolean
  Heading_Control : Subsystem
  Heading_Rate_Map : Subsystem
  Logical Operator : Logic  Operator=OR  AllPortsSameDT=off  OutDataTypeStr=boolean
  Motion_State : Stateflow chart  TreatAsAtomicUnit=on
  Psi_rate_cmd_TD : Subsystem
  Saturation1 : Saturate  UpperLimit=FMS_PARAM.YAW_RATE_LIM  LowerLimit=-FMS_PARAM.YAW_RATE_LIM
  Switch : Switch  Criteria=u2 > Threshold
  move_check : Subsystem
  psi_rate : Subsystem
  psi_rate_cmd_radPs : Outport
  wires:
  Saturation1/1 -> psi_rate_cmd_radPs/1
  Switch/1 -> Psi_rate_cmd_TD/1(v)
  INS_Out/1 -> Heading_Control/2(INS_Out), psi_rate/1(INS_Out)
  move_check/1(move_cmd) -> Motion_State/1(move_cmd)
  psi_rate/1(heading_rate) -> Motion_State/2(heading_rate)
  Compare To Constant/1 -> Switch/2, Detect Increase/1
  FMS_Cmd/1 -> Heading_Rate_Map/2(FMS_Cmd), move_check/1(FMS_Cmd)
  Heading_Rate_Map/1(psi_rate_cmd_radPs) -> Switch/3
  Motion_State/1(state) -> Compare To Constant/1, Heading_Rate_Map/1(state)  "alt_mode_psi_state"
  Logical Operator/1 -> Heading_Control/1(update)
  Heading_Control/1(psi_rate_cmd_radPs) -> Switch/1
  FMS_Out/1 -> Bus Selector/1
  Bus Selector/1 -> Compare To Constant1/1  "<state>"
  Compare To Constant1/1 -> Detect Increase1/1
  Detect Increase1/1 -> Logical Operator/1  "just_arm"
  Detect Increase/1 -> Logical Operator/2
  Psi_rate_cmd_TD/1(v1) -> Saturation1/1

== system old_FMS/Control_Mode/Position_Mode/Command_Generator/Vel_Command ==
  FMS_Cmd : Inport
  INS_Out : Inport  Port=2
  Motion_State : Subsystem
  Subsystem1 : Subsystem
  line_speed : Subsystem
  move_check : Subsystem
  vel_cmd_C_mPs : Outport
  wires:
  Subsystem1/1(vel_cmd_C_mPs) -> vel_cmd_C_mPs/1
  FMS_Cmd/1 -> Subsystem1/1(FMS_Cmd), move_check/1(FMS_Cmd)
  INS_Out/1 -> Subsystem1/3(INS_Out), line_speed/1(INS_Out)
  move_check/1(move_cmd) -> Motion_State/1(move_cmd)
  line_speed/1(ground_speed) -> Motion_State/2(ground_speed)
  line_speed/2(vz) -> Motion_State/3(vz)
  Motion_State/1(motion_state) -> Subsystem1/2(motion_state)

== system old_FMS/Control_Mode/Altitude_Hold_Mode/Command_Generator/Attitude_Command/Phi_CMD_TD ==
  v : Inport
  Integrator : DiscreteIntegrator  SampleTime=-1  ICPrevOutput=DiscIntNeverNeededParam  ICPrevScaledInput=DiscIntNeverNeededParam
  Integrator1 : DiscreteIntegrator  SampleTime=-1  ICPrevOutput=DiscIntNeverNeededParam  ICPrevScaledInput=DiscIntNeverNeededParam
  Subtract : Sum  Inputs=+-
  "fhan " : Subsystem  mask{r0=4*pi, h0=0.04}
      mask DialogControl ParameterGroupVar Prompt: fhan(v1,v2,r0,h0)
  v1 : Outport
  wires:
  Integrator1/1 -> v1/1, Subtract/1
  v/1 -> Subtract/2
  Integrator/1 -> "fhan "/2(v2), Integrator1/1  "v2"
  Subtract/1 -> "fhan "/1(v1)
  "fhan "/1(fhan) -> Integrator/1

== system old_FMS/Control_Mode/Altitude_Hold_Mode/Command_Generator/Attitude_Command/Thera_CMD_TD ==
  v : Inport
  Integrator : DiscreteIntegrator  SampleTime=-1  ICPrevOutput=DiscIntNeverNeededParam  ICPrevScaledInput=DiscIntNeverNeededParam
  Integrator1 : DiscreteIntegrator  SampleTime=-1  ICPrevOutput=DiscIntNeverNeededParam  ICPrevScaledInput=DiscIntNeverNeededParam
  Subtract : Sum  Inputs=+-
  "fhan " : Subsystem  mask{r0=4*pi, h0=0.04}
      mask DialogControl ParameterGroupVar Prompt: fhan(v1,v2,r0,h0)
  v1 : Outport
  wires:
  "fhan "/1(fhan) -> Integrator/1
  Subtract/1 -> "fhan "/1(v1)
  Integrator/1 -> "fhan "/2(v2), Integrator1/1  "v2"
  v/1 -> Subtract/2
  Integrator1/1 -> Subtract/1, v1/1

== system old_FMS/Control_Mode/Altitude_Hold_Mode/Command_Generator/Psi_Rate_Command/Heading_Control ==
  update : Inport
  INS_Out : Inport  Port=2
  Gain2 : Gain  Gain=FMS_PARAM.YAW_P  OutDataTypeStr=single
  Heading_Error : Subsystem
  psi_rate_cmd_radPs : Outport
  wires:
  update/1 -> Heading_Error/2(update)
  INS_Out/1 -> Heading_Error/1(INS_Out)
  Heading_Error/1(psi_err_rad) -> Gain2/1
  Gain2/1 -> psi_rate_cmd_radPs/1

== system old_FMS/Control_Mode/Altitude_Hold_Mode/Command_Generator/Psi_Rate_Command/Heading_Rate_Map ==
  state : Inport
  FMS_Cmd : Inport  Port=2
  Bus Selector : BusSelector  OutputSignals=stick_yaw
  Compare To Constant : simulink/Logic and Bit Operations/Compare To Constant  relop===  const=1  OutDataTypeStr=boolean
  Constant : Constant  Value=0  VectorParams1D=off  OutDataTypeStr=single
  Gain1 : Gain  Gain=FMS_PARAM.YAW_RATE_LIM  OutDataTypeStr=single
  Stretch : Subsystem
  Switch1 : Switch  Criteria=u2 > Threshold
  psi_rate_cmd_radPs : Outport
  wires:
  Constant/1 -> Switch1/1  "brake_speed"
  Switch1/1 -> psi_rate_cmd_radPs/1
  Gain1/1 -> Switch1/3
  state/1 -> Compare To Constant/1
  Compare To Constant/1 -> Switch1/2
  FMS_Cmd/1 -> Bus Selector/1
  Bus Selector/1 -> Stretch/1(u)  "<stick_yaw>"
  Stretch/1(y) -> Gain1/1

== system old_FMS/Control_Mode/Altitude_Hold_Mode/Command_Generator/Psi_Rate_Command/Psi_rate_cmd_TD ==
  v : Inport
  Integrator : DiscreteIntegrator  SampleTime=-1  ICPrevOutput=DiscIntNeverNeededParam  ICPrevScaledInput=DiscIntNeverNeededParam
  Integrator1 : DiscreteIntegrator  SampleTime=-1  ICPrevOutput=DiscIntNeverNeededParam  ICPrevScaledInput=DiscIntNeverNeededParam
  Subtract : Sum  Inputs=+-
  "fhan " : Subsystem  mask{r0=2*pi, h0=0.04}
      mask DialogControl ParameterGroupVar Prompt: fhan(v1,v2,r0,h0)
  v1 : Outport
  wires:
  Integrator1/1 -> v1/1, Subtract/1
  v/1 -> Subtract/2
  Integrator/1 -> "fhan "/2(v2), Integrator1/1  "v2"
  Subtract/1 -> "fhan "/1(v1)
  "fhan "/1(fhan) -> Integrator/1

== system old_FMS/Control_Mode/Altitude_Hold_Mode/Command_Generator/Psi_Rate_Command/move_check ==
  FMS_Cmd : Inport
  Bus Selector : BusSelector  OutputSignals=stick_yaw
  Compare To Zero : simulink/Logic and Bit Operations/Compare To Zero  relop=~=  OutDataTypeStr=boolean
  move_cmd : Outport
  wires:
  FMS_Cmd/1 -> Bus Selector/1
  Compare To Zero/1 -> move_cmd/1
  Bus Selector/1 -> Compare To Zero/1  "<stick_yaw>"

== system old_FMS/Control_Mode/Altitude_Hold_Mode/Command_Generator/Psi_Rate_Command/psi_rate ==
  INS_Out : Inport
  Abs : Abs
  Bus Selector : BusSelector  OutputSignals=r
  heading_rate : Outport
  wires:
  INS_Out/1 -> Bus Selector/1
  Abs/1 -> heading_rate/1
  Bus Selector/1 -> Abs/1  "<r>"

== system old_FMS/Control_Mode/Altitude_Hold_Mode/Command_Generator/Vel_Command/Motion_State ==
  move_cmd : Inport
  vz : Inport  Port=2
  Z_Motion_State : Stateflow chart  TreatAsAtomicUnit=on
  motion_state : Outport
  wires:
  Z_Motion_State/1(state) -> motion_state/1  "alt_mode_motion_state"
  vz/1 -> Z_Motion_State/2(speed)
  move_cmd/1 -> Z_Motion_State/1(move_cmd)

== system old_FMS/Control_Mode/Altitude_Hold_Mode/Command_Generator/Vel_Command/Subsystem1 ==
  FMS_Cmd : Inport
  motion_state : Inport  Port=2
  INS_Out : Inport  Port=3
  Compare To Constant1 : simulink/Logic and Bit Operations/Compare To Constant  relop===  const=2  OutDataTypeStr=boolean
  Height_Control : Subsystem
  Switch1 : Switch  Criteria=u2 > Threshold
  Velocity_Map : Subsystem
  W_CMD_TD : Subsystem
  vel_w_cmd_C_mPs : Outport
  wires:
  Switch1/1 -> W_CMD_TD/1(v)  "w1"
  Velocity_Map/1(vel_w_cmd_C_mPs) -> Switch1/3
  Height_Control/1(vel_w_cmd_C_mPs) -> Switch1/1
  Compare To Constant1/1 -> Switch1/2
  motion_state/1 -> Height_Control/1(motion_state), Compare To Constant1/1, Velocity_Map/1(motion_state)
  FMS_Cmd/1 -> Velocity_Map/2(FMS_Cmd)
  INS_Out/1 -> Height_Control/2(INS_Out)
  W_CMD_TD/1(v1) -> vel_w_cmd_C_mPs/1  "w2"

== system old_FMS/Control_Mode/Altitude_Hold_Mode/Command_Generator/Vel_Command/line_speed ==
  INS_Out : Inport
  Bus Selector : BusSelector  OutputSignals=vd
  vz : Outport
  wires:
  Bus Selector/1 -> vz/1  "<vd>"
  INS_Out/1 -> Bus Selector/1

== system old_FMS/Control_Mode/Altitude_Hold_Mode/Command_Generator/Vel_Command/move_check ==
  FMS_Cmd : Inport
  Bus Selector : BusSelector  OutputSignals=stick_throttle
  Compare To Zero1 : simulink/Logic and Bit Operations/Compare To Zero  relop=~=  OutDataTypeStr=boolean
  move_cmd : Outport
  wires:
  Compare To Zero1/1 -> move_cmd/1
  Bus Selector/1 -> Compare To Zero1/1  "<stick_throttle>"
  FMS_Cmd/1 -> Bus Selector/1

== system old_FMS/Control_Mode/Manual_Mode/Command_Generator/Attitude_Command/Phi_CMD_TD ==
  v : Inport
  Integrator : DiscreteIntegrator  SampleTime=-1  ICPrevOutput=DiscIntNeverNeededParam  ICPrevScaledInput=DiscIntNeverNeededParam
  Integrator1 : DiscreteIntegrator  SampleTime=-1  ICPrevOutput=DiscIntNeverNeededParam  ICPrevScaledInput=DiscIntNeverNeededParam
  Subtract : Sum  Inputs=+-
  "fhan " : Subsystem  mask{r0=4*pi, h0=0.04}
      mask DialogControl ParameterGroupVar Prompt: fhan(v1,v2,r0,h0)
  v1 : Outport
  wires:
  Integrator1/1 -> v1/1, Subtract/1
  v/1 -> Subtract/2
  Integrator/1 -> "fhan "/2(v2), Integrator1/1  "v2"
  Subtract/1 -> "fhan "/1(v1)
  "fhan "/1(fhan) -> Integrator/1

== system old_FMS/Control_Mode/Manual_Mode/Command_Generator/Attitude_Command/Theta_CMD_TD ==
  v : Inport
  Integrator : DiscreteIntegrator  SampleTime=-1  ICPrevOutput=DiscIntNeverNeededParam  ICPrevScaledInput=DiscIntNeverNeededParam
  Integrator1 : DiscreteIntegrator  SampleTime=-1  ICPrevOutput=DiscIntNeverNeededParam  ICPrevScaledInput=DiscIntNeverNeededParam
  Subtract : Sum  Inputs=+-
  "fhan " : Subsystem  mask{r0=4*pi, h0=0.04}
      mask DialogControl ParameterGroupVar Prompt: fhan(v1,v2,r0,h0)
  v1 : Outport
  wires:
  "fhan "/1(fhan) -> Integrator/1
  Subtract/1 -> "fhan "/1(v1)
  Integrator/1 -> "fhan "/2(v2), Integrator1/1  "v2"
  v/1 -> Subtract/2
  Integrator1/1 -> Subtract/1, v1/1

== system old_FMS/Control_Mode/Manual_Mode/Command_Generator/Psi_Rate_Command/Heading_Control ==
  update : Inport
  INS_Out : Inport  Port=2
  Gain2 : Gain  Gain=FMS_PARAM.YAW_P  OutDataTypeStr=single
  Heading_Error : Subsystem
  psi_rate_cmd_radPs : Outport
  wires:
  Gain2/1 -> psi_rate_cmd_radPs/1
  Heading_Error/1(psi_err_rad) -> Gain2/1
  INS_Out/1 -> Heading_Error/1(INS_Out)
  update/1 -> Heading_Error/2(update)

== system old_FMS/Control_Mode/Manual_Mode/Command_Generator/Psi_Rate_Command/Heading_Rate_Map ==
  state : Inport
  FMS_Cmd : Inport  Port=2
  Bus Selector : BusSelector  OutputSignals=stick_yaw
  Compare To Constant : simulink/Logic and Bit Operations/Compare To Constant  relop===  const=1  OutDataTypeStr=boolean
  Constant : Constant  Value=0  VectorParams1D=off  OutDataTypeStr=single
  Gain1 : Gain  Gain=FMS_PARAM.YAW_RATE_LIM  OutDataTypeStr=single
  Stretch : Subsystem
  Switch1 : Switch  Criteria=u2 > Threshold
  psi_rate_cmd_radPs : Outport
  wires:
  Bus Selector/1 -> Stretch/1(u)  "<stick_yaw>"
  FMS_Cmd/1 -> Bus Selector/1
  Compare To Constant/1 -> Switch1/2
  state/1 -> Compare To Constant/1
  Gain1/1 -> Switch1/3
  Switch1/1 -> psi_rate_cmd_radPs/1
  Constant/1 -> Switch1/1  "brake_speed"
  Stretch/1(y) -> Gain1/1

== system old_FMS/Control_Mode/Manual_Mode/Command_Generator/Psi_Rate_Command/move_check ==
  FMS_Cmd : Inport
  Bus Selector : BusSelector  OutputSignals=stick_yaw
  Compare To Zero : simulink/Logic and Bit Operations/Compare To Zero  relop=~=  OutDataTypeStr=boolean
  move_cmd : Outport
  wires:
  Bus Selector/1 -> Compare To Zero/1  "<stick_yaw>"
  Compare To Zero/1 -> move_cmd/1
  FMS_Cmd/1 -> Bus Selector/1

== system old_FMS/Control_Mode/Manual_Mode/Command_Generator/Psi_Rate_Command/psi_rate ==
  INS_Out : Inport
  Abs : Abs
  Bus Selector : BusSelector  OutputSignals=r
  heading_rate : Outport
  wires:
  Bus Selector/1 -> Abs/1  "<r>"
  Abs/1 -> heading_rate/1
  INS_Out/1 -> Bus Selector/1

== system old_FMS/Control_Mode/Position_Mode/Command_Generator/Psi_Rate_Command1/Heading_Control ==
  update : Inport
  INS_Out : Inport  Port=2
  Gain2 : Gain  Gain=FMS_PARAM.YAW_P  OutDataTypeStr=single
  Heading_Error : Subsystem
  psi_rate_cmd_radPs : Outport
  wires:
  update/1 -> Heading_Error/2(update)
  INS_Out/1 -> Heading_Error/1(INS_Out)
  Heading_Error/1(psi_err_rad) -> Gain2/1
  Gain2/1 -> psi_rate_cmd_radPs/1

== system old_FMS/Control_Mode/Position_Mode/Command_Generator/Psi_Rate_Command1/Heading_Rate_Map ==
  state : Inport
  FMS_Cmd : Inport  Port=2
  Bus Selector : BusSelector  OutputSignals=stick_yaw
  Compare To Constant : simulink/Logic and Bit Operations/Compare To Constant  relop===  const=1  OutDataTypeStr=boolean
  Constant : Constant  Value=0  VectorParams1D=off  OutDataTypeStr=single
  Gain1 : Gain  Gain=FMS_PARAM.YAW_RATE_LIM  OutDataTypeStr=single
  Stretch : Subsystem
  Switch1 : Switch  Criteria=u2 > Threshold
  psi_rate_cmd_radPs : Outport
  wires:
  Constant/1 -> Switch1/1  "brake_speed"
  Switch1/1 -> psi_rate_cmd_radPs/1
  Gain1/1 -> Switch1/3
  state/1 -> Compare To Constant/1
  Compare To Constant/1 -> Switch1/2
  FMS_Cmd/1 -> Bus Selector/1
  Bus Selector/1 -> Stretch/1(u)  "<stick_yaw>"
  Stretch/1(y) -> Gain1/1

== system old_FMS/Control_Mode/Position_Mode/Command_Generator/Psi_Rate_Command1/Psi_rate_cmd_TD ==
  v : Inport
  Integrator : DiscreteIntegrator  SampleTime=-1  ICPrevOutput=DiscIntNeverNeededParam  ICPrevScaledInput=DiscIntNeverNeededParam
  Integrator1 : DiscreteIntegrator  SampleTime=-1  ICPrevOutput=DiscIntNeverNeededParam  ICPrevScaledInput=DiscIntNeverNeededParam
  Subtract : Sum  Inputs=+-
  "fhan " : Subsystem  mask{r0=2*pi, h0=0.04}
      mask DialogControl ParameterGroupVar Prompt: fhan(v1,v2,r0,h0)
  v1 : Outport
  wires:
  Integrator1/1 -> v1/1, Subtract/1
  v/1 -> Subtract/2
  Integrator/1 -> "fhan "/2(v2), Integrator1/1  "v2"
  Subtract/1 -> "fhan "/1(v1)
  "fhan "/1(fhan) -> Integrator/1

== system old_FMS/Control_Mode/Position_Mode/Command_Generator/Psi_Rate_Command1/move_check ==
  FMS_Cmd : Inport
  Bus Selector : BusSelector  OutputSignals=stick_yaw
  Compare To Zero : simulink/Logic and Bit Operations/Compare To Zero  relop=~=  OutDataTypeStr=boolean
  move_cmd : Outport
  wires:
  FMS_Cmd/1 -> Bus Selector/1
  Compare To Zero/1 -> move_cmd/1
  Bus Selector/1 -> Compare To Zero/1  "<stick_yaw>"

== system old_FMS/Control_Mode/Position_Mode/Command_Generator/Psi_Rate_Command1/psi_rate ==
  INS_Out : Inport
  Abs : Abs
  Bus Selector : BusSelector  OutputSignals=r
  heading_rate : Outport
  wires:
  INS_Out/1 -> Bus Selector/1
  Abs/1 -> heading_rate/1
  Bus Selector/1 -> Abs/1  "<r>"

== system old_FMS/Control_Mode/Position_Mode/Command_Generator/Vel_Command/Motion_State ==
  move_cmd : Inport
  ground_speed : Inport  Port=2
  vz : Inport  Port=3
  Mux : Mux  Inputs=2
  Selector : Selector  InputPortWidth=2  IndexOptions=Index vector (dialog)  Indices=1  OutputSizes=1
  Selector1 : Selector  InputPortWidth=2  IndexOptions=Index vector (dialog)  Indices=2  OutputSizes=1
  XY_Motion_State : Stateflow chart  TreatAsAtomicUnit=on
  Z_Motion_State : Stateflow chart  TreatAsAtomicUnit=on
  motion_state : Outport
  wires:
  Mux/1 -> motion_state/1  "pos_mode_motion_state"
  Z_Motion_State/1(state) -> Mux/2
  vz/1 -> Z_Motion_State/2(speed)
  Selector1/1 -> Z_Motion_State/1(move_cmd)
  Selector/1 -> XY_Motion_State/1(move_cmd)
  ground_speed/1 -> XY_Motion_State/2(speed)
  XY_Motion_State/1(state) -> Mux/1
  move_cmd/1 -> Selector/1, Selector1/1

== system old_FMS/Control_Mode/Position_Mode/Command_Generator/Vel_Command/Subsystem1 ==
  FMS_Cmd : Inport
  motion_state : Inport  Port=2
  INS_Out : Inport  Port=3
  Bus Selector1 : BusSelector  OutputSignals=M_CO
  Compare To Constant : simulink/Logic and Bit Operations/Compare To Constant  relop===  const=2  OutDataTypeStr=boolean
  Compare To Constant1 : simulink/Logic and Bit Operations/Compare To Constant  relop===  const=2  OutDataTypeStr=boolean
  Mux : Mux  Inputs=2
  Position_Control : Subsystem
  Saturation : Saturate  UpperLimit=FMS_PARAM.VEL_XY_LIM  LowerLimit=-FMS_PARAM.VEL_XY_LIM
  Saturation1 : Saturate  UpperLimit=FMS_PARAM.VEL_Z_LIM  LowerLimit=-FMS_PARAM.VEL_Z_LIM
  Selector : Selector  InputPortWidth=2  IndexOptions=Index vector (dialog)  Indices=1  OutputSizes=1
  Selector1 : Selector  InputPortWidth=2  IndexOptions=Index vector (dialog)  Indices=2  OutputSizes=1
  Switch : Switch  Criteria=u2 > Threshold
  Switch1 : Switch  Criteria=u2 > Threshold
  Velocity_Map : Subsystem
  W_CMD_TD : Subsystem
  vel_cmd_C_mPs : Outport
  wires:
  Mux/1 -> W_CMD_TD/1(v)
  Switch1/1 -> Saturation1/1
  Velocity_Map/2(vel_w_cmd_C_mPs) -> Switch1/3
  Position_Control/2(vel_w_cmd_C_mPs) -> Switch1/1
  Compare To Constant1/1 -> Switch1/2
  Selector1/1 -> Compare To Constant1/1
  motion_state/1 -> Selector/1, Selector1/1, Velocity_Map/1(motion_state), Position_Control/2(motion_state)
  Selector/1 -> Compare To Constant/1
  Velocity_Map/1(vel_uv_cmd_C_mPs) -> Switch/3
  Position_Control/1(vel_uv_cmd_C_mPs) -> Switch/1
  FMS_Cmd/1 -> Velocity_Map/2(FMS_Cmd), Bus Selector1/1
  Switch/1 -> Saturation/1
  Bus Selector1/1 -> Position_Control/1(M_CO)  "<M_CO>"
  INS_Out/1 -> Position_Control/3(INS_Out)
  Compare To Constant/1 -> Switch/2
  Saturation/1 -> Mux/1
  Saturation1/1 -> Mux/2
  W_CMD_TD/1(v1) -> vel_cmd_C_mPs/1

== system old_FMS/Control_Mode/Position_Mode/Command_Generator/Vel_Command/line_speed ==
  INS_Out : Inport
  Add : Sum
  Bus Selector : BusSelector  OutputSignals=vn,ve,vd
  Math Function : Math  Operator=square  SaturateOnIntegerOverflow=on
  Math Function1 : Math  Operator=square  SaturateOnIntegerOverflow=on
  Sqrt : Sqrt  SaturateOnIntegerOverflow=on
  ground_speed : Outport
  vz : Outport  Port=2
  wires:
  Add/1 -> Sqrt/1
  Math Function1/1 -> Add/2
  Math Function/1 -> Add/1
  Sqrt/1 -> ground_speed/1
  Bus Selector/3 -> vz/1  "<vd>"
  Bus Selector/2 -> Math Function1/1  "<ve>"
  Bus Selector/1 -> Math Function/1  "<vn>"
  INS_Out/1 -> Bus Selector/1

== system old_FMS/Control_Mode/Position_Mode/Command_Generator/Vel_Command/move_check ==
  FMS_Cmd : Inport
  Bus Selector : BusSelector  OutputSignals=stick_pitch,stick_roll,stick_throttle
  Compare To Zero : simulink/Logic and Bit Operations/Compare To Zero  relop=~=  OutDataTypeStr=boolean
  Compare To Zero1 : simulink/Logic and Bit Operations/Compare To Zero  relop=~=  OutDataTypeStr=boolean
  Logical Operator : Logic  Operator=OR  Inputs=1  AllPortsSameDT=off  OutDataTypeStr=boolean
  Mux : Mux  Inputs=2
  Mux1 : Mux  Inputs=2
  move_cmd : Outport
  wires:
  Mux1/1 -> move_cmd/1
  Compare To Zero1/1 -> Mux1/2
  Logical Operator/1 -> Mux1/1
  Bus Selector/2 -> Mux/2  "<stick_roll>"
  Bus Selector/1 -> Mux/1  "<stick_pitch>"
  Compare To Zero/1 -> Logical Operator/1
  Mux/1 -> Compare To Zero/1
  Bus Selector/3 -> Compare To Zero1/1  "<stick_throttle>"
  FMS_Cmd/1 -> Bus Selector/1
